simulink model "coupled_tanks"  (R2015b)
settings: Solver=ode1  StartTime=0.0  StopTime=inf  FixedStep=0.002  RelTol=1e-3
PostLoadFcn:
  | qc_set_target_type(getConfigSet(bdroot, 'QUARC Default Target Configuration'));
undefined symbols (not defined in the file): HIL
libraries: simulink x6, quarc_library x3
settings Model: SimulationMode=external  ExtModeTrigDuration=30000  Creator=MLevis  LastModifiedBy=UFRN
settings SolverCC: PositivePriorityOrder=on
settings DataIOCC: SaveFormat=Array  SignalLoggingSaveFormat=ModelDataLogs
settings OptimizationCC: ExpressionDepthLimit=2147483647  InitFltsAndDblsToZero=on
settings DebuggingCC: SaveWithParameterizedLinksMsg=none  UnderspecifiedInitializationDetection=Classic  MergeDetectMultiDrivingBlocksExec=none  SolverPrmCheckMsg=warning  MultiTaskDSMMsg=warning  MultiTaskCondExecSysMsg=none  FcnCallInpInsideContextMsg=UseLocalSettings  StateNameClashWarn=warning
settings HardwareCC: ProdBitPerPointer=32  ProdLargestAtomicFloat=None  ProdIntDivRoundTo=Undefined  ProdEndianess=Unspecified  ProdWordSize=32  ProdHWDeviceType=32-bit Generic
settings RTWCC: SystemTargetFile=quarc_win64.tlc  TemplateMakefile=quarc_default_tmf  Description=QUARC Win64 Target
settings GRTTargetCC: ParMdlRefBuildCompliant=off  CompOptLevelCompliant=off  GeneratePreprocessorConditionals=Disable all  CombineOutputUpdateFcns=off  MatFileLogging=off  GRTInterface=on  UseToolchainInfoCompliant=off  ExtMode=on  ExtModeMexFile=quarc_comm
settings ConfigComp: CovModelRefEnable=Off

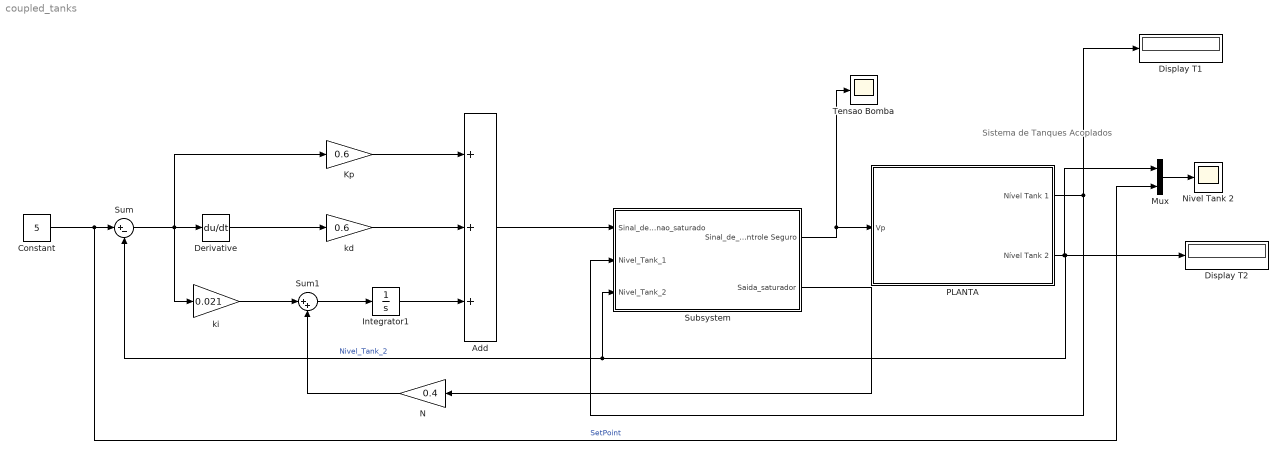
== system coupled_tanks ==
  note: Sistema de Tanques Acoplados
  Add : Sum  Inputs=+++
  Constant : Constant  Value=5
  Derivative : Derivative
  "Display T1 " : Display
  Display T2 : Display
  Integrator1 : Integrator
  Kp : Gain  Gain=0.6
  Mux : Mux  Inputs=2
  "N " : Gain  Gain=0.4
  Nivel Tank 2 : Scope
  PLANTA : Subsystem
  Subsystem : Subsystem
  Sum : Sum  Inputs=|+-
  Sum1 : Sum  Inputs=|++
  Tensao Bomba : Scope
  "kd " : Gain  Gain=0.6
  "ki " : Gain  Gain=0.021
  wires:
  PLANTA/1(Nível Tank 1) -> "Display T1 "/1, Subsystem/2(Nivel_Tank_1)
  Sum/1 -> "ki "/1, Derivative/1, Kp/1
  Constant/1 -> Mux/2, Sum/1  "SetPoint"
  Mux/1 -> Nivel Tank 2/1
  Kp/1 -> Add/1
  Derivative/1 -> "kd "/1
  Add/1 -> Subsystem/1(Sinal_de_controle nao_saturado)
  Subsystem/1(Sinal_de_controle Seguro) -> Tensao Bomba/1, PLANTA/1(Vp)
  PLANTA/2(Nível Tank 2) -> Display T2/1, Sum/2, Subsystem/3(Nivel_Tank_2), Mux/1  "Nivel_Tank_2"
  "kd "/1 -> Add/2
  "ki "/1 -> Sum1/1
  Sum1/1 -> Integrator1/1
  Integrator1/1 -> Add/3
  Subsystem/2("Saida_saturador ") -> "N "/1
  "N "/1 -> Sum1/2

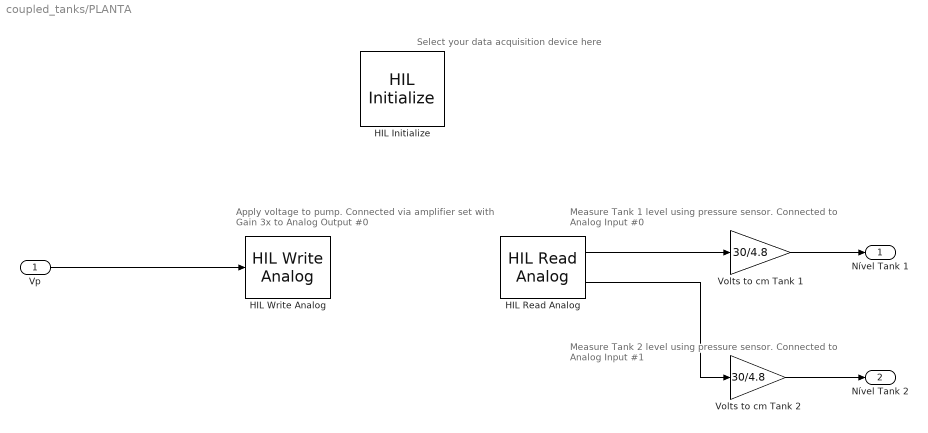
== system coupled_tanks/PLANTA ==
  note: Select your data acquisition device here
  note: Apply voltage to pump.
      | Connected via amplifier set with Gain 3x
      | to  Analog Output #0
  note: Measure Tank 2 level using pressure sensor.
      | Connected to Analog Input #1
  note: Measure Tank 1 level using pressure sensor.
      | Connected to Analog Input #0
  Vp : Inport
  HIL Initialize : quarc_library/Data Acquisition/Generic/Configuration/HIL Initialize  object_name=HIL-1  board_type=q8_usb  board_number=0  board_options=update_rate=normal;decimation=1  exclusive=off  active=off  hardware_clocks=[0:2]  clock_modes=[]  initial_clock_frequencies=[]  set_clock_params_at_start=off  set_clock_params_at_switch_in=off  set_clock_frequencies_at_start=off  set_clock_frequencies_at_switch_in=off  analog_input_channels=[0:7]  analog_input_maximums=10  analog_input_minimums=-10  set_analog_input_params_at_start=on  set_analog_input_params_at_switch_in=off  analog_output_channels=[0:7]  analog_output_maximums=10  analog_output_minimums=-10  initial_analog_outputs=[0]  final_analog_outputs=[0]  watchdog_analog_outputs=0  set_analog_output_params_at_start=on  set_analog_output_params_at_switch_in=off  set_analog_outputs_at_start=on  set_analog_outputs_at_switch_in=off  set_analog_outputs_at_terminate=on  set_analog_outputs_at_switch_out=off  set_analog_outputs_on_watchdog=off  digital_input_channels=[]  digital_output_channels=[]  digital_output_configuration=[]  initial_digital_outputs=[1]  final_digital_outputs=[1]  watchdog_digital_outputs=[1]  set_digital_output_params_at_start=off  set_digital_output_params_at_switch_in=off  set_digital_outputs_at_start=on  set_digital_outputs_at_switch_in=off  set_digital_outputs_at_terminate=on  set_digital_outputs_at_switch_out=off  set_digital_outputs_on_watchdog=off  encoder_channels=[0:7]  quadrature=[4]  encoder_filter_frequency=[]  initial_encoder_counts=[0]  set_encoder_params_at_start=on  set_encoder_params_at_switch_in=off  set_encoder_counts_at_start=on  set_encoder_counts_at_switch_in=off  pwm_channels=[0:7]  pwm_modes=0  pwm_frequency=99.532799999999995e6/4095  pwm_configuration=[0]  pwm_alignment=[0]  pwm_polarity=[1]  pwm_leading_deadband=[0]  pwm_trailing_deadband=[0]  initial_pwm_outputs=[0]  final_pwm_outputs=[0]  watchdog_pwm_outputs=[0]  set_pwm_params_at_start=on  set_pwm_params_at_switch_in=off  set_pwm_outputs_at_start=on  set_pwm_outputs_at_switch_in=off  set_pwm_outputs_at_terminate=on  set_pwm_outputs_at_switch_out=off  set_pwm_outputs_on_watchdog=off  other_output_channels=[]  initial_other_outputs=[]  final_other_outputs=[]  watchdog_other_outputs=[]  set_other_outputs_at_start=off  set_other_outputs_at_switch_in=off  set_other_outputs_at_terminate=off  set_other_outputs_at_switch_out=off  set_other_outputs_on_watchdog=off
  HIL Read Analog : quarc_library/Data Acquisition/Generic/Immediate I//O/HIL Read Analog  object_name=HIL-1  channels=[0:1]  sample_time=qc_get_step_size  active=on  vector_output=off
  HIL Write Analog : quarc_library/Data Acquisition/Generic/Immediate I//O/HIL Write Analog  object_name=HIL-1  channels=0  sample_time=-1  active=off  vector_input=off
  "Volts to cm Tank 1 " : Gain  Gain=30/4.8
  Volts to cm Tank 2 : Gain  Gain=30/4.8
  Nível Tank 1 : Outport
  Nível Tank 2 : Outport  Port=2
  wires:
  HIL Read Analog/1 -> "Volts to cm Tank 1 "/1
  HIL Read Analog/2 -> Volts to cm Tank 2/1
  Vp/1 -> HIL Write Analog/1
  "Volts to cm Tank 1 "/1 -> Nível Tank 1/1
  Volts to cm Tank 2/1 -> Nível Tank 2/1

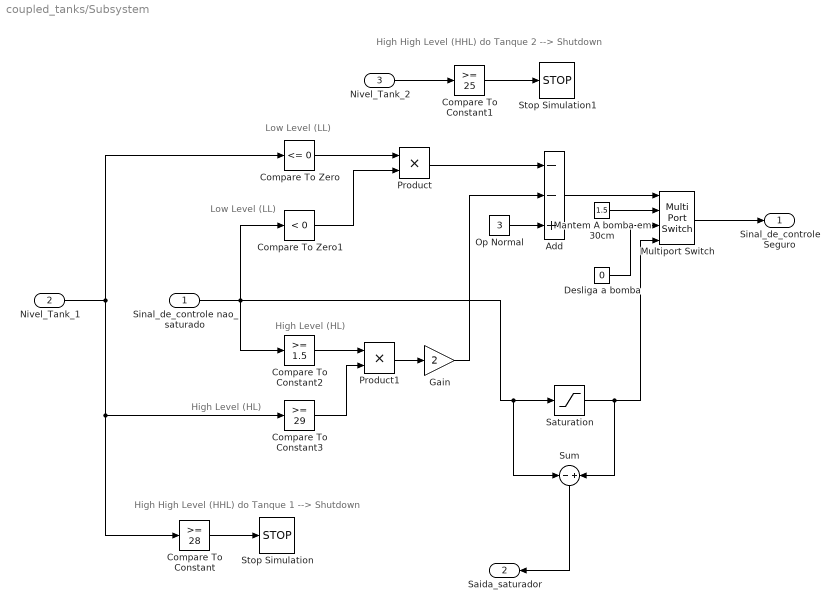
== system coupled_tanks/Subsystem ==
  note: High High Level (HHL) do Tanque 2 --> Shutdown
  note: High High Level (HHL) do Tanque 1 --> Shutdown
  note: Low Level (LL)
  note: Low Level (LL)
  note: High Level (HL)
  note: High Level (HL)
  Sinal_de_controle nao_saturado : Inport
  Nivel_Tank_1 : Inport  Port=2
  Nivel_Tank_2 : Inport  Port=3
  Add : Sum  Inputs=--+
  Compare To Constant : simulink/Logic and Bit Operations/Compare To Constant  relop=>=  const=28  OutDataTypeStr=boolean
  Compare To Constant1 : simulink/Logic and Bit Operations/Compare To Constant  relop=>=  const=25  OutDataTypeStr=boolean
  Compare To Constant2 : simulink/Logic and Bit Operations/Compare To Constant  relop=>=  const=1.5  OutDataTypeStr=boolean
  Compare To Constant3 : simulink/Logic and Bit Operations/Compare To Constant  relop=>=  const=29  OutDataTypeStr=boolean
  Compare To Zero : simulink/Logic and Bit Operations/Compare To Zero  relop=<=  OutDataTypeStr=boolean
  Compare To Zero1 : simulink/Logic and Bit Operations/Compare To Zero  relop=<  OutDataTypeStr=boolean
  Desliga a bomba : Constant  Value=0
  Gain : Gain  Gain=2
  Mantem A bomba em 30cm : Constant  Value=1.5
  Multiport Switch : MultiPortSwitch
  Op Normal : Constant  Value=3
  Product : Product
  Product1 : Product
  Saturation : Saturate  UpperLimit=4  LowerLimit=-4
  Stop Simulation : Stop
  Stop Simulation1 : Stop
  Sum : Sum  Inputs=-|+
  Sinal_de_controle Seguro : Outport
  "Saida_saturador " : Outport  Port=2
  wires:
  Nivel_Tank_1/1 -> Compare To Constant3/1, Compare To Constant/1, Compare To Zero/1
  Compare To Constant/1 -> Stop Simulation/1
  Compare To Zero/1 -> Product/1
  Compare To Zero1/1 -> Product/2
  Multiport Switch/1 -> Sinal_de_controle Seguro/1
  Product/1 -> Add/1
  Saturation/1 -> Sum/2, Multiport Switch/4
  Sinal_de_controle nao_saturado/1 -> Sum/1, Saturation/1, Compare To Constant2/1, Compare To Zero1/1
  Nivel_Tank_2/1 -> Compare To Constant1/1
  Compare To Constant1/1 -> Stop Simulation1/1
  Compare To Constant2/1 -> Product1/1
  Add/1 -> Multiport Switch/1
  Compare To Constant3/1 -> Product1/2
  Product1/1 -> Gain/1
  Gain/1 -> Add/2
  Op Normal/1 -> Add/3
  Mantem A bomba em 30cm/1 -> Multiport Switch/2
  Desliga a bomba/1 -> Multiport Switch/3
  Sum/1 -> "Saida_saturador "/1
